simulink model "BLDCmotor_modeling"  (R2015b)
settings: Solver=VariableStepAuto  StartTime=0.0  StopTime=inf  RelTol=1e-3
values from neighbouring files (symbols this model uses):
  B = 0.1    [BLDCmotor_modeling_param.m]
  J = 0.02    [BLDCmotor_modeling_param.m]
  ke = 0.31    [BLDCmotor_modeling_param.m]
  kt = 0.51    [BLDCmotor_modeling_param.m]
  L = 0.5    [BLDCmotor_modeling_param.m]
  P = 30    [BLDCmotor_modeling_param.m]
  R = 0.02    [BLDCmotor_modeling_param.m]
undefined symbols (not defined in the file or in its folder): trapezoid
settings Model: Creator=weberhsu  LastModifiedBy=shangwei

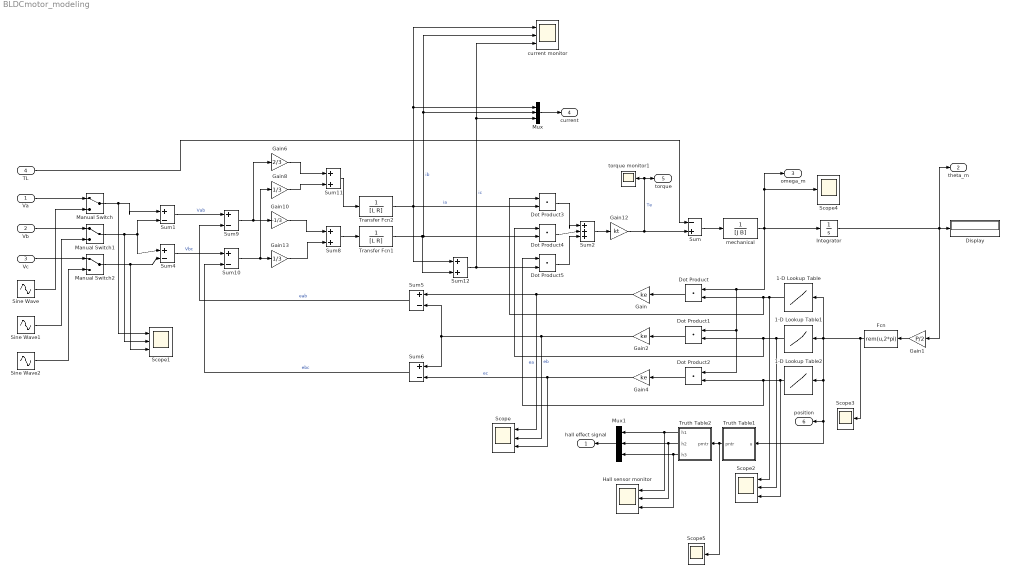
== system BLDCmotor_modeling ==
  Va : Inport
  Vb : Inport  Port=2
  Vc : Inport  Port=3
  TL : Inport  Port=4
  1-D Lookup Table : Lookup_n-D  NumberOfTableDimensions=1  BreakpointsForDimension1=0:0.01:2*pi  Table=trapezoid(0:0.01:2*pi,0)  InternalRulePriority=Speed  RndMeth=Simplest  InputSameDT=on
  1-D Lookup Table1 : Lookup_n-D  NumberOfTableDimensions=1  BreakpointsForDimension1=((0:0.01:2*pi))  Table=trapezoid(0:0.01:2*pi, 2/3*pi)  InternalRulePriority=Speed  RndMeth=Simplest  InputSameDT=on
  1-D Lookup Table2 : Lookup_n-D  NumberOfTableDimensions=1  BreakpointsForDimension1=(0:0.01:2*pi)  Table=trapezoid(0:0.01:2*pi, 4/3*pi)  InternalRulePriority=Speed  RndMeth=Simplest  InputSameDT=on
  Display : Display
  Dot Product{,1..5} (6 alike) : DotProduct  InputSameDT=on  OutDataTypeStr=Inherit: Inherit via internal rule
  Fcn : Fcn  Expr=rem(u,2*pi)
  Gain : Gain  Gain=ke
  Gain1 : Gain  Gain=P/2
  Gain10 : Gain  Gain=-1/3
  Gain12 : Gain  Gain=kt
  Gain13 : Gain  Gain=1/3
  Gain2 : Gain  Gain=ke
  Gain4 : Gain  Gain=ke
  Gain6 : Gain  Gain=2/3
  Gain8 : Gain  Gain=1/3
  Hall sensor monitor : Scope  NumInputPorts=3
  Integrator : Integrator
  Manual Switch : ManualSwitch
  Manual Switch1 : ManualSwitch
  Manual Switch2 : ManualSwitch
  Mux : Mux  Inputs=3
  Mux1 : Mux  Inputs=3
  Scope : Scope  NumInputPorts=3
  Scope1 : Scope  NumInputPorts=3
  Scope2 : Scope  NumInputPorts=3
  Scope3 : Scope
  Scope4 : Scope
  Scope5 : Scope
  Sine Wave : Sin  Amplitude=24  SampleTime=0
  Sine Wave1 : Sin  Amplitude=24  Phase=2/3*pi  SampleTime=0
  Sine Wave2 : Sin  Amplitude=24  Phase=4/3*pi  SampleTime=0
  Sum : Sum  Inputs=-+
  Sum1 : Sum  Inputs=|+-
  Sum{5..6,9..10} (4 alike) : Sum  Inputs=+-
  Sum11 : Sum
  Sum12 : Sum
  Sum2 : Sum  Inputs=|+++
  Sum4 : Sum  Inputs=|+-
  Sum8 : Sum
  Transfer Fcn1 : TransferFcn  Denominator=[L R]
  Transfer Fcn2 : TransferFcn  Denominator=[L R]
  Truth Table1 : Truth Table  TreatAsAtomicUnit=on
  Truth Table2 : Truth Table  TreatAsAtomicUnit=on
  current monitor : Scope  NumInputPorts=3
  mechanical : TransferFcn  Denominator=[J B]
  torque monitor1 : Scope
  hall effect signal : Outport
  theta_m : Outport  Port=2
  omega_m : Outport  Port=3
  current : Outport  Port=4
  torque : Outport  Port=5
  position : Outport  Port=6
  wires:
  Sum/1 -> mechanical/1
  Gain12/1 -> torque/1, torque monitor1/1, Sum/2  "Te"
  Sum2/1 -> Gain12/1
  Dot Product3/1 -> Sum2/1
  Dot Product4/1 -> Sum2/2
  Dot Product5/1 -> Sum2/3
  Sum1/1 -> Sum9/1  "Vab"
  Sum4/1 -> Sum10/1  "Vbc"
  Gain/1 -> Scope/1, Sum5/1  "ea"
  Gain2/1 -> Scope/2, Sum6/1, Sum5/2  "eb"
  Gain4/1 -> Sum6/2, Scope/3  "ec"
  Sum5/1 -> Sum9/2  "eab"
  Sum6/1 -> Sum10/2  "ebc"
  Gain10/1 -> Sum8/1
  Sum8/1 -> Transfer Fcn1/1
  Transfer Fcn1/1 -> Dot Product4/2, current monitor/2, Mux/2, Sum12/2  "ib"
  Sum9/1 -> Gain10/1, Gain6/1
  Sum10/1 -> Gain8/1, Gain13/1
  Transfer Fcn2/1 -> current monitor/1, Mux/1, Dot Product3/2, Sum12/1  "ia"
  Gain6/1 -> Sum11/1
  Gain8/1 -> Sum11/2
  Sum11/1 -> Transfer Fcn2/1
  Sum12/1 -> current monitor/3, Mux/3, Dot Product5/2  "ic"
  Gain13/1 -> Sum8/2
  1-D Lookup Table/1 -> Scope2/1, Dot Product/2, Dot Product3/1
  Dot Product/1 -> Gain/1
  1-D Lookup Table1/1 -> Scope2/2, Dot Product1/2, Dot Product4/1
  Dot Product1/1 -> Gain2/1
  Dot Product2/1 -> Gain4/1
  Gain1/1 -> Fcn/1
  TL/1 -> Sum/1
  Mux/1 -> current/1
  Fcn/1 -> Scope3/1, 1-D Lookup Table2/1, Truth Table1/1(u), position/1, 1-D Lookup Table1/1, 1-D Lookup Table/1
  Truth Table2/1(h1) -> Hall sensor monitor/1, Mux1/1
  Truth Table2/2(h2) -> Hall sensor monitor/2, Mux1/2
  Mux1/1 -> hall effect signal/1
  Truth Table2/3(h3) -> Hall sensor monitor/3, Mux1/3
  Sine Wave/1 -> Manual Switch/2
  Sine Wave1/1 -> Manual Switch1/2
  Sine Wave2/1 -> Manual Switch2/2
  1-D Lookup Table2/1 -> Scope2/3, Dot Product2/2, Dot Product5/1
  Va/1 -> Manual Switch/1
  Manual Switch/1 -> Scope1/1, Sum1/1
  Vb/1 -> Manual Switch1/1
  Manual Switch1/1 -> Scope1/2, Sum4/1, Sum1/2
  Vc/1 -> Manual Switch2/1
  Manual Switch2/1 -> Sum4/2, Scope1/3
  Truth Table1/1(pntr) -> Scope5/1, Truth Table2/1(pmtr)
  Integrator/1 -> theta_m/1, Display/1, Gain1/1
  mechanical/1 -> Integrator/1, Scope4/1, omega_m/1, Dot Product2/1, Dot Product1/1, Dot Product/1

== matlab function BLDCmotor_modeling/Truth Table1 ==
  data: u input; pntr output
function pntr = fcn(u)

aVarTruthTableCondition_1 = false;
aVarTruthTableCondition_2 = false;
aVarTruthTableCondition_3 = false;
aVarTruthTableCondition_4 = false;
aVarTruthTableCondition_5 = false;
aVarTruthTableCondition_6 = false;


% 0 ~ 60

aVarTruthTableCondition_1 = logical(0 <= abs(u) && abs(u) < 1/3*pi);

% 60 ~ 120

aVarTruthTableCondition_2 = logical(1/3*pi <= abs(u) && abs(u) < 2/3*pi);

% 120 ~ 180

aVarTruthTableCondition_3 = logical(2/3*pi <= abs(u) && abs(u) < pi);

% 180 ~ 240

aVarTruthTableCondition_4 = logical(pi <= abs(u) && abs(u) < 4/3*pi);

% 240 ~ 300

aVarTruthTableCondition_5 = logical(4/3*pi <= abs(u) && abs(u) < 5/3*pi);

% 300 ~ 360

aVarTruthTableCondition_6 = logical(5/3*pi <= abs(u) && abs(u) < 2*pi);

if (aVarTruthTableCondition_1 && ~aVarTruthTableCondition_2 && ~aVarTruthTableCondition_3 && ~aVarTruthTableCondition_4 && ~aVarTruthTableCondition_5 && ~aVarTruthTableCondition_6)
    cntr1();
elseif (~aVarTruthTableCondition_1 && aVarTruthTableCondition_2 && ~aVarTruthTableCondition_3 && ~aVarTruthTableCondition_4 && ~aVarTruthTableCondition_5 && ~aVarTruthTableCondition_6)
    cntr2();
elseif (~aVarTruthTableCondition_1 && ~aVarTruthTableCondition_2 && aVarTruthTableCondition_3 && ~aVarTruthTableCondition_4 && ~aVarTruthTableCondition_5 && ~aVarTruthTableCondition_6)
    cntr3();
elseif (~aVarTruthTableCondition_1 && ~aVarTruthTableCondition_2 && ~aVarTruthTableCondition_3 && aVarTruthTableCondition_4 && ~aVarTruthTableCondition_5 && ~aVarTruthTableCondition_6)
    cntr4();
elseif (~aVarTruthTableCondition_1 && ~aVarTruthTableCondition_2 && ~aVarTruthTableCondition_3 && ~aVarTruthTableCondition_4 && aVarTruthTableCondition_5 && ~aVarTruthTableCondition_6)
    cntr5();
elseif (~aVarTruthTableCondition_1 && ~aVarTruthTableCondition_2 && ~aVarTruthTableCondition_3 && ~aVarTruthTableCondition_4 && ~aVarTruthTableCondition_5 && aVarTruthTableCondition_6)
    cntr6();
else % Default
    cntr0();
end

function cntr0()

% counter 0

pntr = 0;

function cntr1()

% counter 1

pntr = 1;

function cntr2()

% counter 2

pntr = 2;

function cntr3()

% counter 3

pntr = 3;

function cntr4()

% counter 4

pntr = 4;

function cntr5()

% counter 5

pntr = 5;

function cntr6()

% counter 6

pntr = 6;

== matlab function BLDCmotor_modeling/Truth Table2 ==
  data: pmtr input; h1 output; h2 output; h3 output
function [h1, h2, h3] = fcn(pmtr)

aVarTruthTableCondition_1 = false;
aVarTruthTableCondition_2 = false;
aVarTruthTableCondition_3 = false;
aVarTruthTableCondition_4 = false;
aVarTruthTableCondition_5 = false;
aVarTruthTableCondition_6 = false;


% 1

aVarTruthTableCondition_1 = logical(pmtr == 1);

% 2

aVarTruthTableCondition_2 = logical(pmtr == 2);

% 3

aVarTruthTableCondition_3 = logical(pmtr == 3);

% 4

aVarTruthTableCondition_4 = logical(pmtr == 4);

% 5

aVarTruthTableCondition_5 = logical(pmtr == 5);

% 6

aVarTruthTableCondition_6 = logical(pmtr == 6);

if (aVarTruthTableCondition_1 && ~aVarTruthTableCondition_2 && ~aVarTruthTableCondition_3 && ~aVarTruthTableCondition_4 && ~aVarTruthTableCondition_5 && ~aVarTruthTableCondition_6)
    state5();
elseif (~aVarTruthTableCondition_1 && aVarTruthTableCondition_2 && ~aVarTruthTableCondition_3 && ~aVarTruthTableCondition_4 && ~aVarTruthTableCondition_5 && ~aVarTruthTableCondition_6)
    state1();
elseif (~aVarTruthTableCondition_1 && ~aVarTruthTableCondition_2 && aVarTruthTableCondition_3 && ~aVarTruthTableCondition_4 && ~aVarTruthTableCondition_5 && ~aVarTruthTableCondition_6)
    state3();
elseif (~aVarTruthTableCondition_1 && ~aVarTruthTableCondition_2 && ~aVarTruthTableCondition_3 && aVarTruthTableCondition_4 && ~aVarTruthTableCondition_5 && ~aVarTruthTableCondition_6)
    state2();
elseif (~aVarTruthTableCondition_1 && ~aVarTruthTableCondition_2 && ~aVarTruthTableCondition_3 && ~aVarTruthTableCondition_4 && aVarTruthTableCondition_5 && ~aVarTruthTableCondition_6)
    state6();
elseif (~aVarTruthTableCondition_1 && ~aVarTruthTableCondition_2 && ~aVarTruthTableCondition_3 && ~aVarTruthTableCondition_4 && ~aVarTruthTableCondition_5 && aVarTruthTableCondition_6)
    state4();
else % Default
    state0();
end

function state0()

% state 0

h1 = false;
h2 = false;
h3 = false;

function state1()

% State 1

h1 = true;
h2 = false;
h3 = false;

function state2()

% State 2

h1 = false;
h2 = true;
h3 = false;

function state3()

% State 3

h1 = true;
h2 = true;
h3 = false;

function state4()

% State 4

h1 = false;
h2 = false;
h3 = true;

function state5()

% State 5

h1 = true;
h2 = false;
h3 = true;

function state6()

% State 6

h1 = false;
h2 = true;
h3 = true;
